simulink model "AmrSimulation"  (R2020a)
settings: Solver=ode1  StartTime=0.0  StopTime=inf  FixedStep=0.001  RelTol=1e-3  EnableMultiTasking=on
undefined symbols (not defined in the file): Accumulator, AMR, MSR_REQUEST
libraries: simulink x18, dspsigops x4
settings Model: Creator=MAC Formula Electric  LastModifiedBy=Harjot
settings OptimizationCC: LifeSpan=inf
settings DebuggingCC: SFUnexpectedBacktrackingDiag=warning  SFNoUnconditionalDefaultTransitionDiag=warning  SFExecutionAtInitializationDiag=none  ArithmeticOperatorsInVariantConditions=warning
settings SFSimCC: SimUseLocalCustomCode=off  CustomCodeUndefinedFunction=UseInterfaceOnly
settings RTWCC: RTWUseLocalCustomCode=off
settings CodeAppCC: StateflowObjectComments=on
settings GRTTargetCC: TargetLangStandard=C89/C90 (ANSI)
settings ConfigComp: CovMetricSettings=dw  CovHtmlReporting=on  CovSaveCumulativeToWorkspaceVar=on  CovSaveSingleToWorkspaceVar=on  CovExternalEMLEnable=off

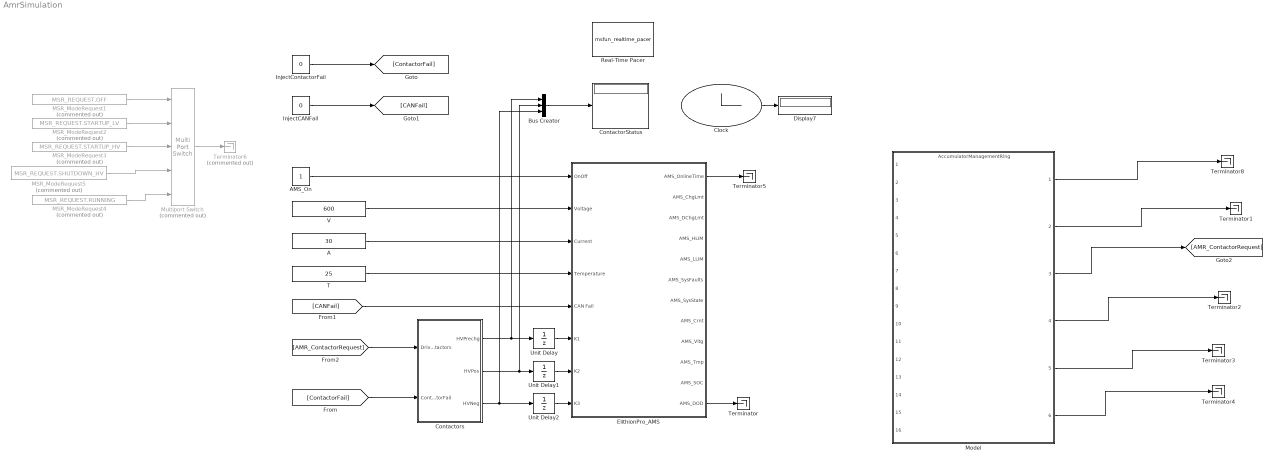
== system AmrSimulation ==
  A : Constant  Value=30
  AMS_On : Constant
  Bus Creator : BusCreator  Inputs=3
  Clock : Clock
  ContactorStatus : Display
  Contactors : Subsystem
  Display7 : Display
  ElithionPro_AMS : Subsystem
  InjectCANFail : Constant  Value=0
  InjectContactorFail : Constant  Value=0
  MSR_ModeRequest1 : Constant  Commented=on  Value=MSR_REQUEST.OFF
  MSR_ModeRequest2 : Constant  Commented=on  Value=MSR_REQUEST.STARTUP_LV
  MSR_ModeRequest3 : Constant  Commented=on  Value=MSR_REQUEST.STARTUP_HV
  MSR_ModeRequest4 : Constant  Commented=on  Value=MSR_REQUEST.RUNNING
  MSR_ModeRequest5 : Constant  Commented=on  Value=MSR_REQUEST.SHUTDOWN_HV
  Model : ModelReference  ModelNameDialog=AccumulatorManagementRing.slx  SimulationMode=Normal  ModelReferenceVersion=1.70
  Multiport Switch : MultiPortSwitch  Commented=on  DataPortOrder=Zero-based contiguous  Inputs=4  zeroidx=on  OutDataTypeStr=Inherit: Inherit via back propagation
      settings: LockScale=on
  Real-Time Pacer : M-S-Function  FunctionName=msfun_realtime_pacer  Parameters=simTimePerRealTime  mask(RealTime_Pacer){simTimePerRealTime=1}
      mask prompts: simTimePerRealTime "Speedup (Simulation Time / Real Time):"
      mask help:
      | Slow down a simulation to track real (i.e., wall clock) elapsed time.
      |
      | "Speedup" specifies the ratio between simulation time and real time
      | • Speedup = N => N sec. of simulation time per sec. of real time
      | • Speedup can be fractional (e.g., 0.5, 1.3).
      | • Speedup = inf => allow simulation to run at full speed
      |
      | Click on the Help button for details.
      mask Help: web('realtime_pacer_help.html', '-helpbrowser')
      mask Display: fprintf('Real-Time Pacer\nSpeedup = %g', simTimePerRealTime)
  T : Constant  Value=25
  Terminator{,1..5,8} (7 alike) : Terminator
  Terminator6 : Terminator  Commented=on
  Unit Delay : UnitDelay  SampleTime=-1  HasFrameUpgradeWarning=on
  Unit Delay1 : UnitDelay  SampleTime=-1  HasFrameUpgradeWarning=on
  Unit Delay2 : UnitDelay  SampleTime=-1  HasFrameUpgradeWarning=on
  V : Constant  Value=600
  wires:
  Model/2 -> Terminator1/1
  Model/3 -> [AMR_ContactorRequest]
  AMS_On/1 -> ElithionPro_AMS/1(OnOff)
  Contactors/1(HVPrechg) -> Bus Creator/1, Unit Delay/1
  Contactors/2(HVPos) -> Bus Creator/2, Unit Delay1/1
  Unit Delay/1 -> ElithionPro_AMS/6(K1)
  Unit Delay1/1 -> ElithionPro_AMS/7(K2)
  Unit Delay2/1 -> ElithionPro_AMS/8(K3)
  InjectContactorFail/1 -> [ContactorFail]
  InjectCANFail/1 -> [CANFail]
  [ContactorFail] -> Contactors/2(ContactorFail)
  [AMR_ContactorRequest] -> Contactors/1(DriveContactors)
  Bus Creator/1 -> ContactorStatus/1
  Clock/1 -> Display7/1
  [CANFail] -> ElithionPro_AMS/5(CAN Fail)
  V/1 -> ElithionPro_AMS/2(Voltage)
  A/1 -> ElithionPro_AMS/3(Current)
  T/1 -> ElithionPro_AMS/4(Temperature)
  ElithionPro_AMS/12(AMS_DOD) -> Terminator/1
  Contactors/3(HVNeg) -> Bus Creator/3, Unit Delay2/1
  Model/4 -> Terminator2/1
  Model/5 -> Terminator3/1
  Model/6 -> Terminator4/1
  Model/1 -> Terminator8/1
  MSR_ModeRequest1/1 -> Multiport Switch/1
  MSR_ModeRequest2/1 -> Multiport Switch/2
  MSR_ModeRequest3/1 -> Multiport Switch/3
  MSR_ModeRequest5/1 -> Multiport Switch/4
  ElithionPro_AMS/1(AMS_OnlineTime) -> Terminator5/1
  MSR_ModeRequest4/1 -> Multiport Switch/5
  Multiport Switch/1 -> Terminator6/1

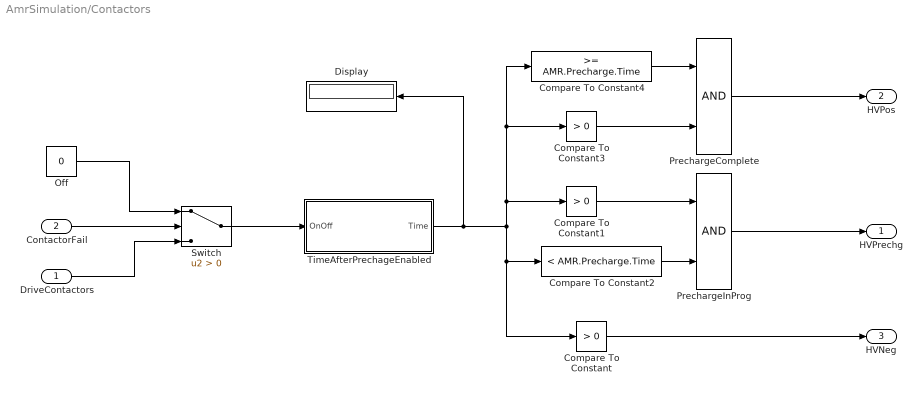
== system AmrSimulation/Contactors ==
  DriveContactors : Inport
  ContactorFail : Inport  Port=2
  Compare To Constant : simulink/Logic and Bit Operations/Compare To Constant  relop=>  const=0  OutDataTypeStr=boolean
  Compare To Constant1 : simulink/Logic and Bit Operations/Compare To Constant  relop=>  const=0  OutDataTypeStr=boolean
  Compare To Constant2 : simulink/Logic and Bit Operations/Compare To Constant  relop=<  const=AMR.Precharge.Time  OutDataTypeStr=boolean
  Compare To Constant3 : simulink/Logic and Bit Operations/Compare To Constant  relop=>  const=0  OutDataTypeStr=boolean
  Compare To Constant4 : simulink/Logic and Bit Operations/Compare To Constant  relop=>=  const=AMR.Precharge.Time  OutDataTypeStr=boolean
  Display : Display
  Off : Constant  Value=0
  PrechargeComplete : Logic  AllPortsSameDT=off  OutDataTypeStr=boolean
  PrechargeInProg : Logic  AllPortsSameDT=off  OutDataTypeStr=boolean
  Switch : Switch  Criteria=u2 > Threshold
  TimeAfterPrechageEnabled : Subsystem
  HVPrechg : Outport  VectorParamsAs1DForOutWhenUnconnected=off
  HVPos : Outport  Port=2  VectorParamsAs1DForOutWhenUnconnected=off
  HVNeg : Outport  Port=3  VectorParamsAs1DForOutWhenUnconnected=off
  wires:
  PrechargeComplete/1 -> HVPos/1
  Compare To Constant1/1 -> PrechargeInProg/1
  Compare To Constant/1 -> HVNeg/1
  PrechargeInProg/1 -> HVPrechg/1
  Compare To Constant2/1 -> PrechargeInProg/2
  TimeAfterPrechageEnabled/1(Time) -> Display/1, Compare To Constant/1, Compare To Constant2/1, Compare To Constant4/1, Compare To Constant3/1, Compare To Constant1/1
  Switch/1 -> TimeAfterPrechageEnabled/1(OnOff)
  ContactorFail/1 -> Switch/2
  Off/1 -> Switch/1
  DriveContactors/1 -> Switch/3
  Compare To Constant3/1 -> PrechargeComplete/2
  Compare To Constant4/1 -> PrechargeComplete/1

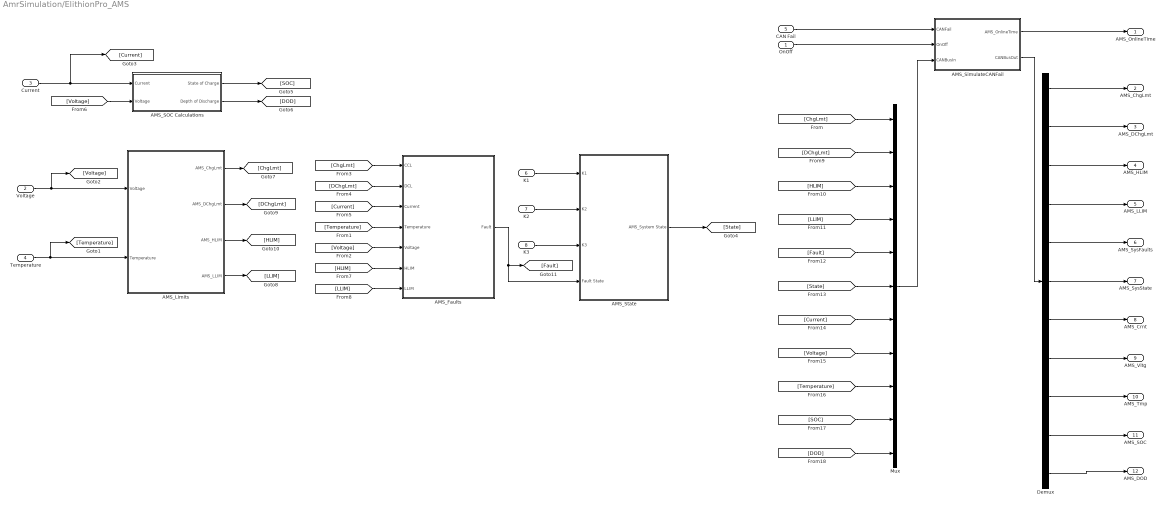
== system AmrSimulation/ElithionPro_AMS ==
  OnOff : Inport
  Voltage : Inport  Port=2
  Current : Inport  Port=3
  Temperature : Inport  Port=4
  CAN Fail : Inport  Port=5
  K1 : Inport  Port=6
  K2 : Inport  Port=7
  K3 : Inport  Port=8
  AMS_Faults : Subsystem
  AMS_Limits : Subsystem
  AMS_SOC Calculations : Subsystem
  AMS_SimulateCANFail : Subsystem
  AMS_State : Subsystem
  Demux : Demux  Outputs=11
  Mux : Mux  Inputs=11
  AMS_OnlineTime : Outport  VectorParamsAs1DForOutWhenUnconnected=off
  AMS_ChgLmt : Outport  Port=2  VectorParamsAs1DForOutWhenUnconnected=off
  AMS_DChgLmt : Outport  Port=3  VectorParamsAs1DForOutWhenUnconnected=off
  AMS_HLIM : Outport  Port=4  VectorParamsAs1DForOutWhenUnconnected=off
  AMS_LLIM : Outport  Port=5  VectorParamsAs1DForOutWhenUnconnected=off
  AMS_SysFaults : Outport  Port=6  VectorParamsAs1DForOutWhenUnconnected=off
  AMS_SysState : Outport  Port=7  VectorParamsAs1DForOutWhenUnconnected=off
  AMS_Crnt : Outport  Port=8  VectorParamsAs1DForOutWhenUnconnected=off
  AMS_Vltg : Outport  Port=9  VectorParamsAs1DForOutWhenUnconnected=off
  AMS_Tmp : Outport  Port=10  VectorParamsAs1DForOutWhenUnconnected=off
  AMS_SOC : Outport  Port=11  VectorParamsAs1DForOutWhenUnconnected=off
  AMS_DOD : Outport  Port=12  VectorParamsAs1DForOutWhenUnconnected=off
  wires:
  Demux/11 -> AMS_DOD/1
  Demux/10 -> AMS_SOC/1
  Demux/9 -> AMS_Tmp/1
  Demux/8 -> AMS_Vltg/1
  Demux/7 -> AMS_Crnt/1
  Demux/6 -> AMS_SysState/1
  Demux/5 -> AMS_SysFaults/1
  Demux/4 -> AMS_LLIM/1
  Demux/3 -> AMS_HLIM/1
  Demux/2 -> AMS_DChgLmt/1
  Demux/1 -> AMS_ChgLmt/1
  AMS_SimulateCANFail/2(CANBusOut) -> Demux/1
  [DOD] -> Mux/11
  [SOC] -> Mux/10
  [Temperature] -> Mux/9
  [Voltage] -> Mux/8
  [Current] -> Mux/7
  [State] -> Mux/6
  [Fault] -> Mux/5
  [ChgLmt] -> Mux/1
  [LLIM] -> Mux/4
  [DChgLmt] -> Mux/2
  [HLIM] -> Mux/3
  Mux/1 -> AMS_SimulateCANFail/3(CANBusIn)
  AMS_SimulateCANFail/1(AMS_OnlineTime) -> AMS_OnlineTime/1
  AMS_State/1(AMS_System State) -> [State]
  [HLIM] -> AMS_Faults/6(HLIM)
  [LLIM] -> AMS_Faults/7(LLIM)
  AMS_Limits/3(AMS_HLIM) -> [HLIM]
  AMS_Limits/2(AMS_DChgLmt) -> [DChgLmt]
  AMS_Limits/1(AMS_ChgLmt) -> [ChgLmt]
  AMS_SOC Calculations/2(Depth of Discharge) -> [DOD]
  AMS_SOC Calculations/1(State of Charge) -> [SOC]
  K3/1 -> AMS_State/3(K3)
  K2/1 -> AMS_State/2(K2)
  K1/1 -> AMS_State/1(K1)
  [Voltage] -> AMS_SOC Calculations/2(Voltage)
  [Voltage] -> AMS_Faults/5(Voltage)
  [ChgLmt] -> AMS_Faults/1(CCL)
  [Current] -> AMS_Faults/3(Current)
  [DChgLmt] -> AMS_Faults/2(DCL)
  [Temperature] -> AMS_Faults/4(Temperature)
  Voltage/1 -> [Voltage], AMS_Limits/1(Voltage)
  Current/1 -> AMS_SOC Calculations/1(Current), [Current]
  Temperature/1 -> [Temperature], AMS_Limits/2(Temperature)
  AMS_Limits/4(AMS_LLIM) -> [LLIM]
  OnOff/1 -> AMS_SimulateCANFail/2(OnOff)
  AMS_Faults/1(Fault) -> AMS_State/4(Fault State), [Fault]
  CAN Fail/1 -> AMS_SimulateCANFail/1(CANFail)

== system AmrSimulation/Contactors/TimeAfterPrechageEnabled ==
  OnOff : Inport
  Discrete Timer : Subsystem
      mask DialogControl Container6 Prompt: Discrete Timer Block
      mask DialogControl Control3 Prompt: This block implements a timer with a reset
  Logical Operator : Logic  Operator=NOT  Inputs=1  AllPortsSameDT=off  OutDataTypeStr=boolean
  Time : Outport  VectorParamsAs1DForOutWhenUnconnected=off
  wires:
  Discrete Timer/1(Time) -> Time/1
  Logical Operator/1 -> Discrete Timer/1(Reset)
  OnOff/1 -> Logical Operator/1

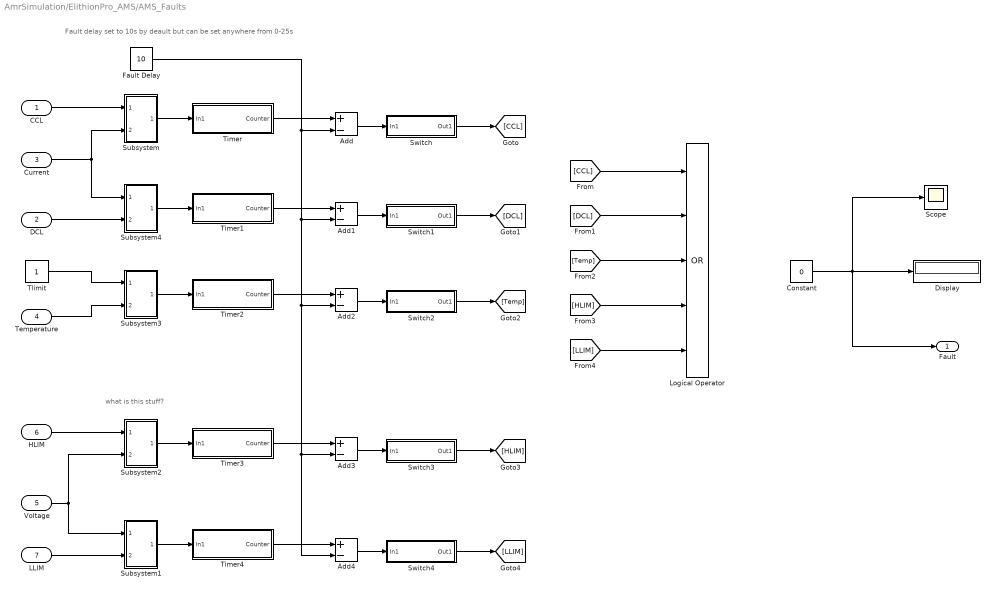
== system AmrSimulation/ElithionPro_AMS/AMS_Faults ==
  note: Fault delay set to 10s by deault but can be set anywhere from 0-25s
  note: what is this stuff?
  CCL : Inport
  DCL : Inport  Port=2
  Current : Inport  Port=3
  Temperature : Inport  Port=4
  Voltage : Inport  Port=5
  HLIM : Inport  Port=6
  LLIM : Inport  Port=7
  Add{,1..4} (5 alike) : Sum  Inputs=+-
  Constant : Constant  Value=0
  Display : Display
  Fault Delay : Constant  Value=10
  Logical Operator : Logic  Operator=OR  Inputs=5  AllPortsSameDT=off  OutDataTypeStr=boolean
  Scope : Scope
  Subsystem : Subsystem
  Subsystem1 : Subsystem
  Subsystem2 : Subsystem
  Subsystem3 : Subsystem
  Subsystem4 : Subsystem
  Switch : Subsystem
  Switch1 : Subsystem
  Switch2 : Subsystem
  Switch3 : Subsystem
  Switch4 : Subsystem
  Timer : Subsystem
  Timer1 : Subsystem
  Timer2 : Subsystem
  Timer3 : Subsystem
  Timer4 : Subsystem
  Tlimit : Constant
  Fault : Outport  VectorParamsAs1DForOutWhenUnconnected=off
  wires:
  Constant/1 -> Display/1, Fault/1, Scope/1
  Add3/1 -> Switch3/1(In1)
  Fault Delay/1 -> Add1/2, Add2/2, Add3/2, Add4/2, Add/2
  Switch2/1(Out1) -> [Temp]
  Subsystem4/1(Out1) -> Timer1/1(In1)
  Switch4/1(Out1) -> [LLIM]
  Subsystem2/1(Out1) -> Timer3/1(In1)
  Add1/1 -> Switch1/1(In1)
  Subsystem1/1(Out1) -> Timer4/1(In1)
  Add2/1 -> Switch2/1(In1)
  Timer3/1(Counter) -> Add3/1
  Timer1/1(Counter) -> Add1/1
  Add4/1 -> Switch4/1(In1)
  Switch3/1(Out1) -> [HLIM]
  Timer4/1(Counter) -> Add4/1
  Timer2/1(Counter) -> Add2/1
  Add/1 -> Switch/1(In1)
  Switch/1(Out1) -> [CCL]
  Switch1/1(Out1) -> [DCL]
  Subsystem3/1(Out1) -> Timer2/1(In1)
  Current/1 -> Subsystem4/1(In1), Subsystem/2(Ibatt)
  Timer/1(Counter) -> Add/1
  CCL/1 -> Subsystem/1(CCL)
  DCL/1 -> Subsystem4/2(In2)
  Temperature/1 -> Subsystem3/2(In2)
  [LLIM] -> Logical Operator/5
  Tlimit/1 -> Subsystem3/1(In1)
  [Temp] -> Logical Operator/3
  Voltage/1 -> Subsystem1/1(In1), Subsystem2/2(In2)
  HLIM/1 -> Subsystem2/1(In1)
  LLIM/1 -> Subsystem1/2(In2)
  [DCL] -> Logical Operator/2
  [HLIM] -> Logical Operator/4
  [CCL] -> Logical Operator/1
  Subsystem/1(Out1) -> Timer/1(In1)

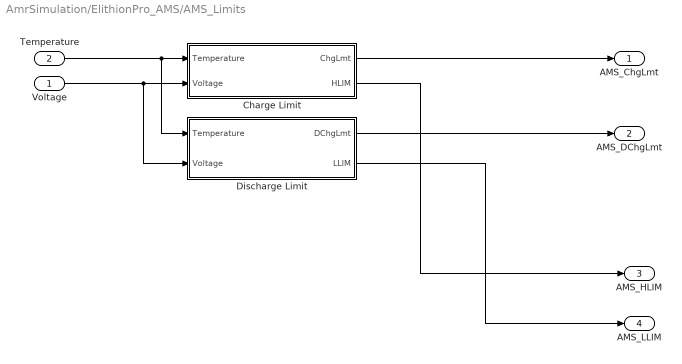
== system AmrSimulation/ElithionPro_AMS/AMS_Limits ==
  Voltage : Inport
  Temperature : Inport  Port=2
  Charge Limit : Subsystem
  Discharge Limit : Subsystem
  AMS_ChgLmt : Outport  VectorParamsAs1DForOutWhenUnconnected=off
  AMS_DChgLmt : Outport  Port=2  VectorParamsAs1DForOutWhenUnconnected=off
  AMS_HLIM : Outport  Port=3  VectorParamsAs1DForOutWhenUnconnected=off
  AMS_LLIM : Outport  Port=4  VectorParamsAs1DForOutWhenUnconnected=off
  wires:
  Voltage/1 -> Discharge Limit/2(Voltage), Charge Limit/2(Voltage)
  Temperature/1 -> Discharge Limit/1(Temperature), Charge Limit/1(Temperature)
  Charge Limit/1(ChgLmt) -> AMS_ChgLmt/1
  Discharge Limit/1(DChgLmt) -> AMS_DChgLmt/1
  Discharge Limit/2(LLIM) -> AMS_LLIM/1
  Charge Limit/2(HLIM) -> AMS_HLIM/1

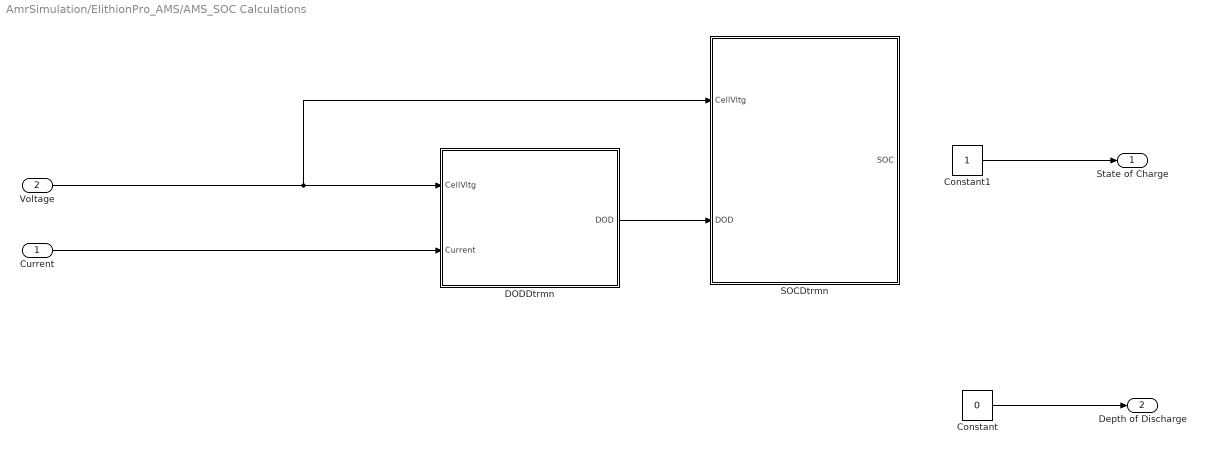
== system AmrSimulation/ElithionPro_AMS/AMS_SOC Calculations ==
  Current : Inport
  Voltage : Inport  Port=2
  Constant : Constant  Value=0
  Constant1 : Constant
  DODDtrmn : Subsystem
  SOCDtrmn : Subsystem
  State of Charge : Outport  VectorParamsAs1DForOutWhenUnconnected=off
  Depth of Discharge : Outport  Port=2  VectorParamsAs1DForOutWhenUnconnected=off
  wires:
  Voltage/1 -> DODDtrmn/1(CellVltg), SOCDtrmn/1(CellVltg)
  DODDtrmn/1(DOD) -> SOCDtrmn/2(DOD)
  Current/1 -> DODDtrmn/2(Current)
  Constant/1 -> Depth of Discharge/1
  Constant1/1 -> State of Charge/1

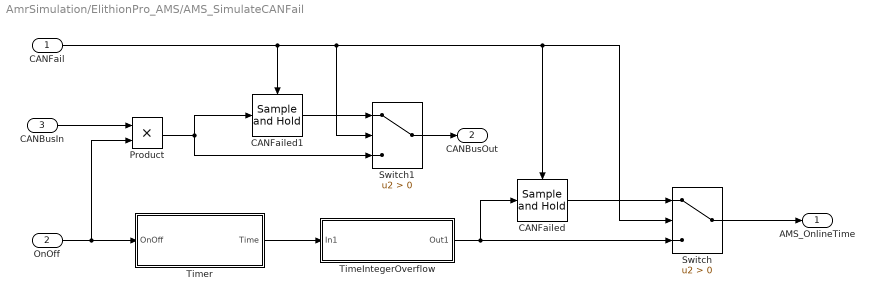
== system AmrSimulation/ElithionPro_AMS/AMS_SimulateCANFail ==
  CANFail : Inport
  OnOff : Inport  Port=2
  CANBusIn : Inport  Port=3
  CANFailed : dspsigops/Sample and Hold  trig=Rising edge  initCond=0  latchinput=off
  CANFailed1 : dspsigops/Sample and Hold  trig=Rising edge  initCond=0  latchinput=off
  Product : Product
  Switch : Switch  Criteria=u2 > Threshold
  Switch1 : Switch  Criteria=u2 > Threshold
  TimeIntegerOverflow : Subsystem
  Timer : Subsystem
  AMS_OnlineTime : Outport  VectorParamsAs1DForOutWhenUnconnected=off
  CANBusOut : Outport  Port=2  VectorParamsAs1DForOutWhenUnconnected=off
  wires:
  Product/1 -> CANFailed1/1, Switch1/3
  CANBusIn/1 -> Product/1
  Switch/1 -> AMS_OnlineTime/1
  CANFailed/1 -> Switch/1
  CANFail/1 -> Switch1/2, CANFailed/Trigger, Switch/2, CANFailed1/Trigger
  Timer/1(Time) -> TimeIntegerOverflow/1(In1)
  TimeIntegerOverflow/1(Out1) -> Switch/3, CANFailed/1
  OnOff/1 -> Timer/1(OnOff), Product/2
  Switch1/1 -> CANBusOut/1
  CANFailed1/1 -> Switch1/1

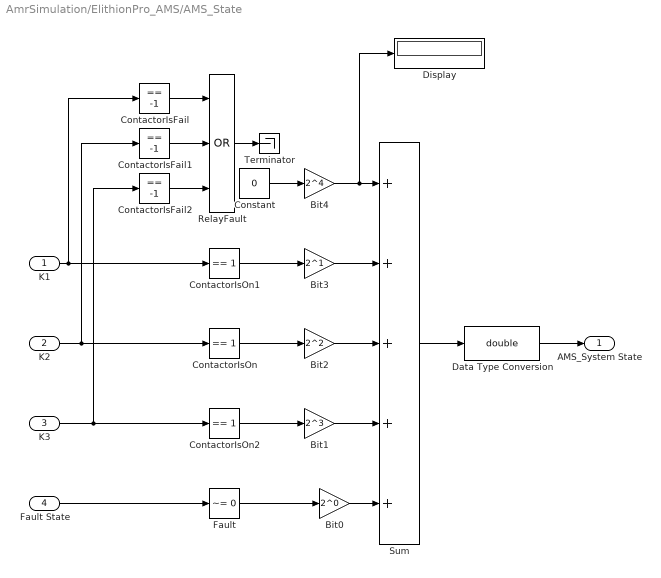
== system AmrSimulation/ElithionPro_AMS/AMS_State ==
  K1 : Inport
  K2 : Inport  Port=2
  K3 : Inport  Port=3
  Fault State : Inport  Port=4
  Bit0 : Gain  Gain=2^0
  Bit1 : Gain  Gain=2^3
  Bit2 : Gain  Gain=2^2
  Bit3 : Gain  Gain=2^1
  Bit4 : Gain  Gain=2^4
  Constant : Constant  Value=0
  ContactorIsFail : simulink/Logic and Bit Operations/Compare To Constant  relop===  const=-1  OutDataTypeStr=boolean
  ContactorIsFail1 : simulink/Logic and Bit Operations/Compare To Constant  relop===  const=-1  OutDataTypeStr=boolean
  ContactorIsFail2 : simulink/Logic and Bit Operations/Compare To Constant  relop===  const=-1  OutDataTypeStr=boolean
  ContactorIsOn : simulink/Logic and Bit Operations/Compare To Constant  relop===  const=1  OutDataTypeStr=boolean
  ContactorIsOn1 : simulink/Logic and Bit Operations/Compare To Constant  relop===  const=1  OutDataTypeStr=boolean
  ContactorIsOn2 : simulink/Logic and Bit Operations/Compare To Constant  relop===  const=1  OutDataTypeStr=boolean
  Data Type Conversion : DataTypeConversion  OutDataTypeStr=double
  Display : Display
  Fault : simulink/Logic and Bit Operations/Compare To Zero  relop=~=  OutDataTypeStr=boolean
  RelayFault : Logic  Operator=OR  Inputs=3  AllPortsSameDT=off  OutDataTypeStr=boolean
  Sum : Sum  Inputs=5  OutDataTypeStr=int8
  Terminator : Terminator
  AMS_System State : Outport  VectorParamsAs1DForOutWhenUnconnected=off
  wires:
  Sum/1 -> Data Type Conversion/1
  Bit0/1 -> Sum/5
  Bit1/1 -> Sum/4
  Bit2/1 -> Sum/3
  Bit3/1 -> Sum/2
  Bit4/1 -> Display/1, Sum/1
  ContactorIsFail2/1 -> RelayFault/3
  ContactorIsFail1/1 -> RelayFault/2
  ContactorIsFail/1 -> RelayFault/1
  K3/1 -> ContactorIsOn2/1, ContactorIsFail2/1
  K2/1 -> ContactorIsOn/1, ContactorIsFail1/1
  K1/1 -> ContactorIsOn1/1, ContactorIsFail/1
  Fault State/1 -> Fault/1
  ContactorIsOn1/1 -> Bit3/1
  ContactorIsOn/1 -> Bit2/1
  ContactorIsOn2/1 -> Bit1/1
  Fault/1 -> Bit0/1
  Data Type Conversion/1 -> AMS_System State/1
  RelayFault/1 -> Terminator/1
  Constant/1 -> Bit4/1

== system AmrSimulation/Contactors/TimeAfterPrechageEnabled/Discrete Timer ==
  Reset : Inport
  Compare To Constant : simulink/Logic and Bit Operations/Compare To Constant  relop=<  const=1  OutDataTypeStr=boolean
  Constant : Constant  Value=0
  Switch : Switch  Criteria=u2 ~= 0
  Unit Delay : UnitDelay  SampleTime=-1  HasFrameUpgradeWarning=on
  Weighted Sample Time : SampleTimeMath
  Time : Outport  VectorParamsAs1DForOutWhenUnconnected=off
  wires:
  Unit Delay/1 -> Switch/1
  Switch/1 -> Time/1, Weighted Sample Time/1
  Compare To Constant/1 -> Switch/2
  Reset/1 -> Compare To Constant/1
  Constant/1 -> Switch/3
  Weighted Sample Time/1 -> Unit Delay/1

== system AmrSimulation/ElithionPro_AMS/AMS_Faults/Subsystem ==
  CCL : Inport
  Ibatt : Inport  Port=2
  Add : Sum  Inputs=+-
  False : Constant  Value=0
  Switch : Switch  Criteria=u2 > Threshold
  True : Constant
  Out1 : Outport  VectorParamsAs1DForOutWhenUnconnected=off
  wires:
  False/1 -> Switch/1
  Add/1 -> Switch/2
  Switch/1 -> Out1/1
  CCL/1 -> Add/1
  Ibatt/1 -> Add/2
  True/1 -> Switch/3

== system AmrSimulation/ElithionPro_AMS/AMS_Faults/Subsystem1 ==
  In1 : Inport
  In2 : Inport  Port=2
  Add4 : Sum  Inputs=+-
  False4 : Constant  Value=0
  Switch4 : Switch  Criteria=u2 > Threshold
  True4 : Constant
  Out1 : Outport  VectorParamsAs1DForOutWhenUnconnected=off
  wires:
  Add4/1 -> Switch4/2
  Switch4/1 -> Out1/1
  True4/1 -> Switch4/3
  False4/1 -> Switch4/1
  In2/1 -> Add4/1
  In1/1 -> Add4/2

== system AmrSimulation/ElithionPro_AMS/AMS_Faults/Subsystem2 ==
  In1 : Inport
  In2 : Inport  Port=2
  Add3 : Sum  Inputs=+-
  False3 : Constant  Value=0
  Switch3 : Switch  Criteria=u2 > Threshold
  True3 : Constant
  Out1 : Outport  VectorParamsAs1DForOutWhenUnconnected=off
  wires:
  Add3/1 -> Switch3/2
  Switch3/1 -> Out1/1
  True3/1 -> Switch3/3
  In1/1 -> Add3/1
  False3/1 -> Switch3/1
  In2/1 -> Add3/2

== system AmrSimulation/ElithionPro_AMS/AMS_Faults/Subsystem3 ==
  In1 : Inport
  In2 : Inport  Port=2
  Add2 : Sum  Inputs=+-
  False2 : Constant  Value=0
  Switch2 : Switch  Criteria=u2 > Threshold
  True2 : Constant
  Out1 : Outport  VectorParamsAs1DForOutWhenUnconnected=off
  wires:
  Add2/1 -> Switch2/2
  True2/1 -> Switch2/3
  Switch2/1 -> Out1/1
  False2/1 -> Switch2/1
  In1/1 -> Add2/1
  In2/1 -> Add2/2

== system AmrSimulation/ElithionPro_AMS/AMS_Faults/Subsystem4 ==
  In1 : Inport
  In2 : Inport  Port=2
  Add1 : Sum  Inputs=+-
  False1 : Constant  Value=0
  Switch1 : Switch  Criteria=u2 > Threshold
  True1 : Constant
  Out1 : Outport  VectorParamsAs1DForOutWhenUnconnected=off
  wires:
  Switch1/1 -> Out1/1
  In1/1 -> Add1/1
  True1/1 -> Switch1/3
  False1/1 -> Switch1/1
  Add1/1 -> Switch1/2
  In2/1 -> Add1/2

== system AmrSimulation/ElithionPro_AMS/AMS_Faults/Switch ==
  In1 : Inport
  Constant : Constant
  Constant1 : Constant  Value=0
  Switch : Switch  Criteria=u2 > Threshold
  Out1 : Outport  VectorParamsAs1DForOutWhenUnconnected=off
  wires:
  Constant/1 -> Switch/1
  In1/1 -> Switch/2
  Constant1/1 -> Switch/3
  Switch/1 -> Out1/1

== system AmrSimulation/ElithionPro_AMS/AMS_Faults/Switch1 ==
  In1 : Inport
  Constant : Constant
  Constant1 : Constant  Value=0
  Switch : Switch  Criteria=u2 > Threshold
  Out1 : Outport  VectorParamsAs1DForOutWhenUnconnected=off
  wires:
  Switch/1 -> Out1/1
  Constant1/1 -> Switch/3
  In1/1 -> Switch/2
  Constant/1 -> Switch/1

== system AmrSimulation/ElithionPro_AMS/AMS_Faults/Switch2 ==
  In1 : Inport
  Constant : Constant
  Constant1 : Constant  Value=0
  Switch : Switch  Criteria=u2 > Threshold
  Out1 : Outport  VectorParamsAs1DForOutWhenUnconnected=off
  wires:
  Constant/1 -> Switch/1
  In1/1 -> Switch/2
  Constant1/1 -> Switch/3
  Switch/1 -> Out1/1

== system AmrSimulation/ElithionPro_AMS/AMS_Faults/Switch3 ==
  In1 : Inport
  Constant : Constant
  Constant1 : Constant  Value=0
  Switch : Switch  Criteria=u2 > Threshold
  Out1 : Outport  VectorParamsAs1DForOutWhenUnconnected=off
  wires:
  Switch/1 -> Out1/1
  Constant1/1 -> Switch/3
  In1/1 -> Switch/2
  Constant/1 -> Switch/1

== system AmrSimulation/ElithionPro_AMS/AMS_Faults/Switch4 ==
  In1 : Inport
  Constant : Constant
  Constant1 : Constant  Value=0
  Switch : Switch  Criteria=u2 > Threshold
  Out1 : Outport  VectorParamsAs1DForOutWhenUnconnected=off
  wires:
  Constant/1 -> Switch/1
  In1/1 -> Switch/2
  Constant1/1 -> Switch/3
  Switch/1 -> Out1/1

== system AmrSimulation/ElithionPro_AMS/AMS_Faults/Timer ==
  In1 : Inport
  CounterBlock : Subsystem
  Display1 : Display
  Counter : Outport  VectorParamsAs1DForOutWhenUnconnected=off
  wires:
  CounterBlock/1(Counter) -> Display1/1, Counter/1
  In1/1 -> CounterBlock/1(Enable)

== system AmrSimulation/ElithionPro_AMS/AMS_Faults/Timer1 ==
  In1 : Inport
  CounterBlock : Subsystem
  Counter : Outport  VectorParamsAs1DForOutWhenUnconnected=off
  wires:
  In1/1 -> CounterBlock/1(Enable)
  CounterBlock/1(Counter) -> Counter/1

== system AmrSimulation/ElithionPro_AMS/AMS_Faults/Timer2 ==
  In1 : Inport
  CounterBlock : Subsystem
  Display1 : Display
  Counter : Outport  VectorParamsAs1DForOutWhenUnconnected=off
  wires:
  CounterBlock/1(Counter) -> Display1/1, Counter/1
  In1/1 -> CounterBlock/1(Enable)

== system AmrSimulation/ElithionPro_AMS/AMS_Faults/Timer3 ==
  In1 : Inport
  CounterBlock : Subsystem
  Display1 : Display
  Counter : Outport  VectorParamsAs1DForOutWhenUnconnected=off
  wires:
  In1/1 -> CounterBlock/1(Enable)
  CounterBlock/1(Counter) -> Counter/1, Display1/1

== system AmrSimulation/ElithionPro_AMS/AMS_Faults/Timer4 ==
  In1 : Inport
  CounterBlock : Subsystem
  Display1 : Display
  Counter : Outport  VectorParamsAs1DForOutWhenUnconnected=off
  wires:
  CounterBlock/1(Counter) -> Display1/1, Counter/1
  In1/1 -> CounterBlock/1(Enable)

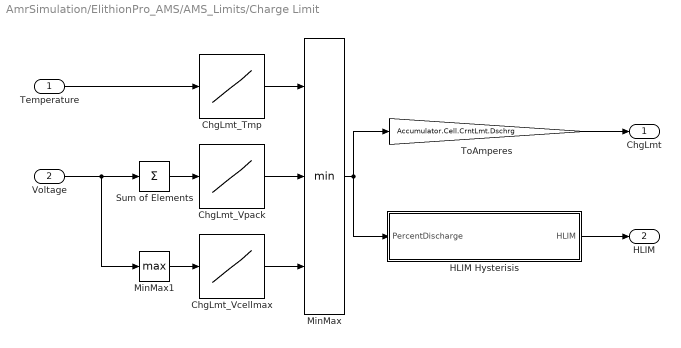
== system AmrSimulation/ElithionPro_AMS/AMS_Limits/Charge Limit ==
  Temperature : Inport
  Voltage : Inport  Port=2
  ChgLmt_Tmp : Lookup_n-D  NumberOfTableDimensions=1  BreakpointsForDimension1=[AMR.Lmt.TChgMin AMR.Lmt.TChgLow AMR.Lmt.TChgHi AMR.Lmt.TChgMax]  Table=[0 1 1 0]  InternalRulePriority=Speed  RndMeth=Simplest  InputSameDT=on
  ChgLmt_Vcellmax : Lookup_n-D  NumberOfTableDimensions=1  BreakpointsForDimension1=[AMR.Lmt.VCellHigh AMR.Lmt.VCellMax]  Table=[1 0]  InternalRulePriority=Speed  RndMeth=Simplest  InputSameDT=on
  ChgLmt_Vpack : Lookup_n-D  NumberOfTableDimensions=1  BreakpointsForDimension1=[AMR.Lmt.VPackHigh AMR.Lmt.VPackMax]  Table=[1 0]  InternalRulePriority=Speed  RndMeth=Simplest  InputSameDT=on
  HLIM Hysterisis : Subsystem
  MinMax : MinMax  Inputs=3
  MinMax1 : MinMax  Function=max
  Sum of Elements : Sum  Inputs=+
  ToAmperes : Gain  Gain=Accumulator.Cell.CrntLmt.Dschrg
  ChgLmt : Outport  VectorParamsAs1DForOutWhenUnconnected=off
  HLIM : Outport  Port=2  VectorParamsAs1DForOutWhenUnconnected=off
  wires:
  Temperature/1 -> ChgLmt_Tmp/1
  Voltage/1 -> MinMax1/1, Sum of Elements/1
  ChgLmt_Tmp/1 -> MinMax/1
  ChgLmt_Vpack/1 -> MinMax/2
  MinMax/1 -> ToAmperes/1, HLIM Hysterisis/1(PercentDischarge)
  HLIM Hysterisis/1(HLIM) -> HLIM/1
  ToAmperes/1 -> ChgLmt/1
  ChgLmt_Vcellmax/1 -> MinMax/3
  MinMax1/1 -> ChgLmt_Vcellmax/1
  Sum of Elements/1 -> ChgLmt_Vpack/1

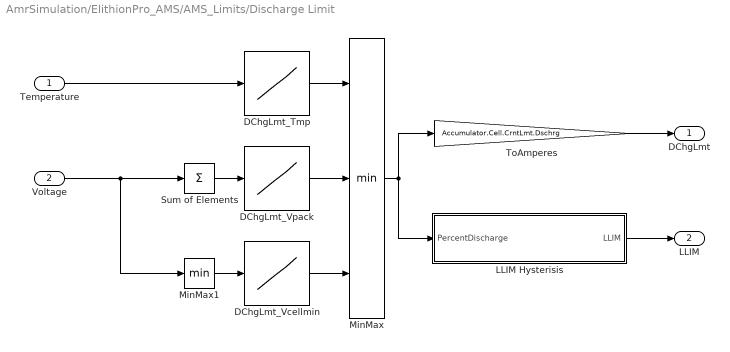
== system AmrSimulation/ElithionPro_AMS/AMS_Limits/Discharge Limit ==
  Temperature : Inport
  Voltage : Inport  Port=2
  DChgLmt_Tmp : Lookup_n-D  NumberOfTableDimensions=1  BreakpointsForDimension1=[AMR.Lmt.TChgMin AMR.Lmt.TChgLow AMR.Lmt.TChgHi AMR.Lmt.TChgMax]  Table=[0 1 1 0]  InternalRulePriority=Speed  RndMeth=Simplest  InputSameDT=on
  DChgLmt_Vcellmin : Lookup_n-D  NumberOfTableDimensions=1  BreakpointsForDimension1=[AMR.Lmt.VCellMin AMR.Lmt.VCellLow]  Table=[0 1]  InternalRulePriority=Speed  RndMeth=Simplest  InputSameDT=on
  DChgLmt_Vpack : Lookup_n-D  NumberOfTableDimensions=1  BreakpointsForDimension1="[AMR.Lmt.VPackMin  AMR.Lmt.VPackLow]"  Table=[0 1]  InternalRulePriority=Speed  RndMeth=Simplest  InputSameDT=on
  LLIM Hysterisis : Subsystem
  MinMax : MinMax  Inputs=3
  MinMax1 : MinMax
  Sum of Elements : Sum  Inputs=+
  ToAmperes : Gain  Gain=Accumulator.Cell.CrntLmt.Dschrg
  DChgLmt : Outport  VectorParamsAs1DForOutWhenUnconnected=off
  LLIM : Outport  Port=2  VectorParamsAs1DForOutWhenUnconnected=off
  wires:
  DChgLmt_Tmp/1 -> MinMax/1
  MinMax/1 -> ToAmperes/1, LLIM Hysterisis/1(PercentDischarge)
  LLIM Hysterisis/1(LLIM) -> LLIM/1
  ToAmperes/1 -> DChgLmt/1
  Temperature/1 -> DChgLmt_Tmp/1
  Voltage/1 -> MinMax1/1, Sum of Elements/1
  MinMax1/1 -> DChgLmt_Vcellmin/1
  Sum of Elements/1 -> DChgLmt_Vpack/1
  DChgLmt_Vpack/1 -> MinMax/2
  DChgLmt_Vcellmin/1 -> MinMax/3

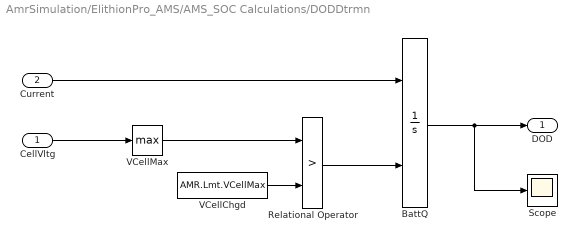
== system AmrSimulation/ElithionPro_AMS/AMS_SOC Calculations/DODDtrmn ==
  CellVltg : Inport
  Current : Inport  Port=2
  BattQ : Integrator  ExternalReset=rising
  Relational Operator : RelationalOperator  Operator=>  OutDataTypeStr=boolean  RndMeth=Nearest
  Scope : Scope
  VCellChgd : Constant  Value=AMR.Lmt.VCellMax
  VCellMax : MinMax  Function=max
  DOD : Outport  VectorParamsAs1DForOutWhenUnconnected=off
  wires:
  VCellMax/1 -> Relational Operator/1
  Current/1 -> BattQ/1
  CellVltg/1 -> VCellMax/1
  VCellChgd/1 -> Relational Operator/2
  BattQ/1 -> DOD/1, Scope/1
  Relational Operator/1 -> BattQ/2

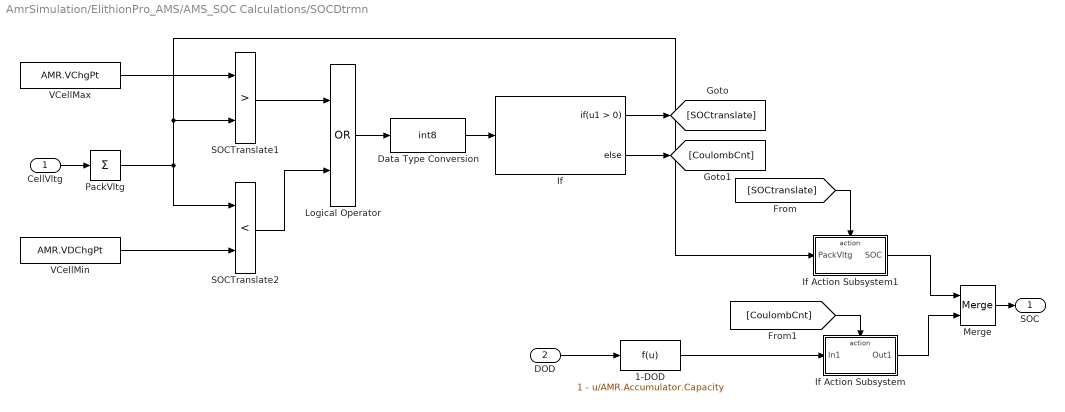
== system AmrSimulation/ElithionPro_AMS/AMS_SOC Calculations/SOCDtrmn ==
  CellVltg : Inport
  DOD : Inport  Port=2
  1-DOD : Fcn  Expr=1 - u/AMR.Accumulator.Capacity
  Data Type Conversion : DataTypeConversion  OutDataTypeStr=int8
  If : If
  If Action Subsystem : Subsystem  TreatAsAtomicUnit=on
  If Action Subsystem1 : Subsystem  TreatAsAtomicUnit=on
  Logical Operator : Logic  Operator=OR  AllPortsSameDT=off  OutDataTypeStr=boolean
  Merge : Merge
  PackVltg : Sum  Inputs=+
  SOCTranslate1 : RelationalOperator  Operator=>  OutDataTypeStr=boolean  RndMeth=Nearest
  SOCTranslate2 : RelationalOperator  Operator=<  OutDataTypeStr=boolean  RndMeth=Nearest
  VCellMax : Constant  Value=AMR.VChgPt
  "VCellMin " : Constant  Value=AMR.VDChgPt
  SOC : Outport  VectorParamsAs1DForOutWhenUnconnected=off
  wires:
  [CoulombCnt] -> If Action Subsystem/Action
  If/2 -> [CoulombCnt]
  If Action Subsystem1/1(SOC) -> Merge/1
  [SOCtranslate] -> If Action Subsystem1/Action
  If/1 -> [SOCtranslate]
  Logical Operator/1 -> Data Type Conversion/1
  SOCTranslate2/1 -> Logical Operator/2
  SOCTranslate1/1 -> Logical Operator/1
  PackVltg/1 -> SOCTranslate2/1, SOCTranslate1/2, If Action Subsystem1/1(PackVltg)
  CellVltg/1 -> PackVltg/1
  DOD/1 -> 1-DOD/1
  1-DOD/1 -> If Action Subsystem/1(In1)
  If Action Subsystem/1(Out1) -> Merge/2
  VCellMax/1 -> SOCTranslate1/1
  "VCellMin "/1 -> SOCTranslate2/2
  Merge/1 -> SOC/1
  Data Type Conversion/1 -> If/1

== system AmrSimulation/ElithionPro_AMS/AMS_SimulateCANFail/TimeIntegerOverflow ==
  note: In the Elithion, this overflows at 2^16
  In1 : Inport
  Display : Display
  Math Function : Math  Operator=mod  SignedPower=on  SaturateOnIntegerOverflow=on
  OverflowTime : Constant  Value=10
  Out1 : Outport  VectorParamsAs1DForOutWhenUnconnected=off
  wires:
  OverflowTime/1 -> Math Function/2
  In1/1 -> Math Function/1
  Math Function/1 -> Out1/1, Display/1

== system AmrSimulation/ElithionPro_AMS/AMS_SimulateCANFail/Timer ==
  OnOff : Inport
  Discrete Timer : Subsystem  AncestorBlock=MFESimulinkLib/Discrete Timer
      mask DialogControl Container6 Prompt: Discrete Timer Block
      mask DialogControl Control3 Prompt: This block implements a timer with a reset
  Logical Operator : Logic  Operator=NOT  Inputs=1  AllPortsSameDT=off  OutDataTypeStr=boolean
  Time : Outport  VectorParamsAs1DForOutWhenUnconnected=off
  wires:
  Discrete Timer/1(Time) -> Time/1
  Logical Operator/1 -> Discrete Timer/1(Reset)
  OnOff/1 -> Logical Operator/1

== system AmrSimulation/ElithionPro_AMS/AMS_Faults/Timer/CounterBlock ==
  Enable : Inport
  Constant : Constant  Value=0
  Memory : Memory
  Product : Product
  Switch : Switch  Criteria=u2 ~= 0
  Weighted Sample Time : SampleTimeMath
  Counter : Outport  VectorParamsAs1DForOutWhenUnconnected=off
  wires:
  Product/1 -> Counter/1
  Constant/1 -> Switch/3
  Memory/1 -> Switch/1
  Enable/1 -> Product/2, Switch/2
  Weighted Sample Time/1 -> Product/1, Memory/1
  Switch/1 -> Weighted Sample Time/1

== system AmrSimulation/ElithionPro_AMS/AMS_Faults/Timer1/CounterBlock ==
  Enable : Inport
  Constant : Constant  Value=0
  Memory : Memory
  Product : Product
  Switch : Switch  Criteria=u2 ~= 0
  Weighted Sample Time : SampleTimeMath
  Counter : Outport  VectorParamsAs1DForOutWhenUnconnected=off
  wires:
  Switch/1 -> Weighted Sample Time/1
  Weighted Sample Time/1 -> Memory/1, Product/1
  Enable/1 -> Switch/2, Product/2
  Memory/1 -> Switch/1
  Constant/1 -> Switch/3
  Product/1 -> Counter/1

== system AmrSimulation/ElithionPro_AMS/AMS_Faults/Timer2/CounterBlock ==
  Enable : Inport
  Constant : Constant  Value=0
  Memory : Memory
  Product : Product
  Switch : Switch  Criteria=u2 ~= 0
  Weighted Sample Time : SampleTimeMath
  Counter : Outport  VectorParamsAs1DForOutWhenUnconnected=off
  wires:
  Product/1 -> Counter/1
  Constant/1 -> Switch/3
  Memory/1 -> Switch/1
  Enable/1 -> Product/2, Switch/2
  Weighted Sample Time/1 -> Product/1, Memory/1
  Switch/1 -> Weighted Sample Time/1

== system AmrSimulation/ElithionPro_AMS/AMS_Faults/Timer3/CounterBlock ==
  Enable : Inport
  Constant : Constant  Value=0
  Memory : Memory
  Product : Product
  Switch : Switch  Criteria=u2 ~= 0
  Weighted Sample Time : SampleTimeMath
  Counter : Outport  VectorParamsAs1DForOutWhenUnconnected=off
  wires:
  Switch/1 -> Weighted Sample Time/1
  Weighted Sample Time/1 -> Memory/1, Product/1
  Enable/1 -> Switch/2, Product/2
  Memory/1 -> Switch/1
  Constant/1 -> Switch/3
  Product/1 -> Counter/1

== system AmrSimulation/ElithionPro_AMS/AMS_Faults/Timer4/CounterBlock ==
  Enable : Inport
  Constant : Constant  Value=0
  Memory : Memory
  Product : Product
  Switch : Switch  Criteria=u2 ~= 0
  Weighted Sample Time : SampleTimeMath
  Counter : Outport  VectorParamsAs1DForOutWhenUnconnected=off
  wires:
  Product/1 -> Counter/1
  Constant/1 -> Switch/3
  Memory/1 -> Switch/1
  Enable/1 -> Product/2, Switch/2
  Weighted Sample Time/1 -> Product/1, Memory/1
  Switch/1 -> Weighted Sample Time/1

== system AmrSimulation/ElithionPro_AMS/AMS_Limits/Charge Limit/HLIM Hysterisis ==
  PercentDischarge : Inport
  Compare To Constant : simulink/Logic and Bit Operations/Compare To Constant  relop===  const=1  OutDataTypeStr=boolean
  Compare To Constant1 : simulink/Logic and Bit Operations/Compare To Constant  relop===  const=0  OutDataTypeStr=boolean
  LLIM_SH : dspsigops/Sample and Hold  trig=Rising edge  initCond=1  latchinput=off
  Logical Operator : Logic  Operator=OR  AllPortsSameDT=off  OutDataTypeStr=boolean
  HLIM : Outport  VectorParamsAs1DForOutWhenUnconnected=off
  wires:
  Compare To Constant1/1 -> Logical Operator/1
  Compare To Constant/1 -> Logical Operator/2
  Logical Operator/1 -> LLIM_SH/Trigger
  LLIM_SH/1 -> HLIM/1
  PercentDischarge/1 -> Compare To Constant1/1, Compare To Constant/1, LLIM_SH/1

== system AmrSimulation/ElithionPro_AMS/AMS_Limits/Discharge Limit/LLIM Hysterisis ==
  PercentDischarge : Inport
  Compare To Constant : simulink/Logic and Bit Operations/Compare To Constant  relop===  const=1  OutDataTypeStr=boolean
  Compare To Constant1 : simulink/Logic and Bit Operations/Compare To Constant  relop===  const=0  OutDataTypeStr=boolean
  LLIM_SH : dspsigops/Sample and Hold  trig=Rising edge  initCond=1  latchinput=off
  Logical Operator : Logic  Operator=OR  AllPortsSameDT=off  OutDataTypeStr=boolean
  LLIM : Outport  VectorParamsAs1DForOutWhenUnconnected=off
  wires:
  Compare To Constant1/1 -> Logical Operator/1
  Compare To Constant/1 -> Logical Operator/2
  Logical Operator/1 -> LLIM_SH/Trigger
  LLIM_SH/1 -> LLIM/1
  PercentDischarge/1 -> Compare To Constant1/1, Compare To Constant/1, LLIM_SH/1

== system AmrSimulation/ElithionPro_AMS/AMS_SOC Calculations/SOCDtrmn/If Action Subsystem ==
  In1 : Inport
  Action Port : ActionPort  ActionPortLabel=else
  Out1 : Outport  VectorParamsAs1DForOutWhenUnconnected=off
  wires:
  In1/1 -> Out1/1

== system AmrSimulation/ElithionPro_AMS/AMS_SOC Calculations/SOCDtrmn/If Action Subsystem1 ==
  PackVltg : Inport
  Action Port : ActionPort  ActionPortLabel=if(u1 > 0)
  1-D Lookup Table : Lookup_n-D  NumberOfTableDimensions=1  BreakpointsForDimension1=[2 3.2 3.3 3.8]  Table=[100 85 3 0]  InternalRulePriority=Speed  RndMeth=Simplest  InputSameDT=on
  SOC : Outport  VectorParamsAs1DForOutWhenUnconnected=off
  wires:
  1-D Lookup Table/1 -> SOC/1
  PackVltg/1 -> 1-D Lookup Table/1

== system AmrSimulation/ElithionPro_AMS/AMS_SimulateCANFail/Timer/Discrete Timer ==
  Reset : Inport
  Compare To Constant : simulink/Logic and Bit Operations/Compare To Constant  relop=<  const=1  OutDataTypeStr=boolean
  Constant : Constant  Value=0
  Switch : Switch  Criteria=u2 ~= 0
  Unit Delay : UnitDelay  SampleTime=-1  HasFrameUpgradeWarning=on
  Weighted Sample Time : SampleTimeMath
  Time : Outport  VectorParamsAs1DForOutWhenUnconnected=off
  wires:
  Unit Delay/1 -> Switch/1
  Switch/1 -> Time/1, Weighted Sample Time/1
  Compare To Constant/1 -> Switch/2
  Reset/1 -> Compare To Constant/1
  Constant/1 -> Switch/3
  Weighted Sample Time/1 -> Unit Delay/1
